simulink model "mac_simulink"  (R2025b)
settings: Solver=VariableStepAuto  StartTime=0.0  StopTime=39  RelTol=1e-3
libraries: hdlsllib x8
settings Model: Creator=aherrman  LastModifiedBy=aherrman

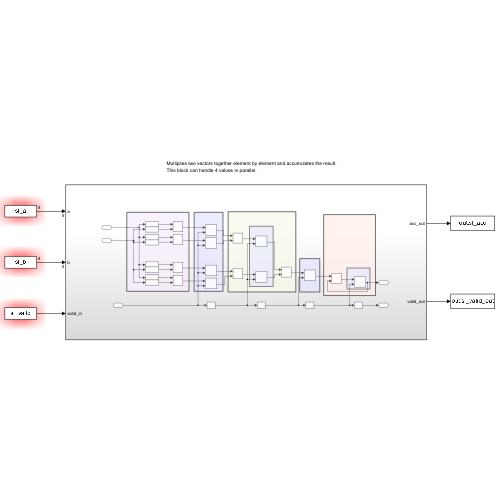
[thumbnail: Simulink's stored preview of the top-level diagram]
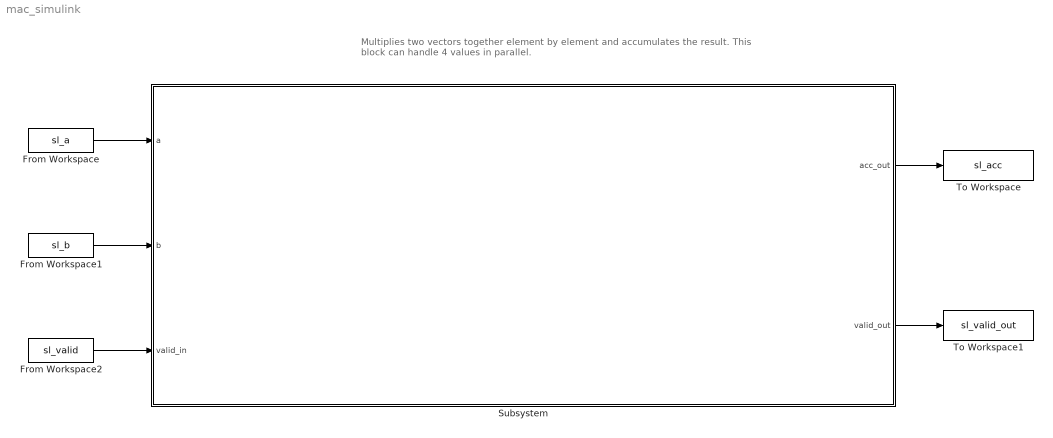
== system mac_simulink ==
  note: Multiplies two vectors together element by element and accumulates the result.
      | This block can handle 4 values in parallel.
  From Workspace : FromWorkspace  VariableName=sl_a  SampleTime=1  OutputAfterFinalValue=Setting to zero
  From Workspace1 : FromWorkspace  VariableName=sl_b  SampleTime=1  OutputAfterFinalValue=Setting to zero
  From Workspace2 : FromWorkspace  VariableName=sl_valid  SampleTime=1  OutputAfterFinalValue=Setting to zero
  Subsystem : Subsystem
  To Workspace : ToWorkspace  VariableName=sl_acc  SaveFormat=Timeseries  SampleTime=-1
  To Workspace1 : ToWorkspace  VariableName=sl_valid_out  SaveFormat=Timeseries  SampleTime=-1
  wires:
  From Workspace/1 -> Subsystem/1(a)
  From Workspace1/1 -> Subsystem/2(b)
  Subsystem/1(acc_out) -> To Workspace/1
  Subsystem/2(valid_out) -> To Workspace1/1
  From Workspace2/1 -> Subsystem/3(valid_in)

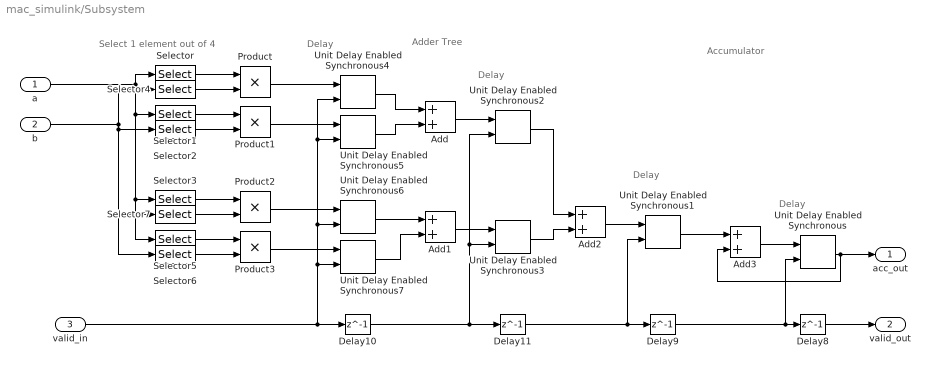
== system mac_simulink/Subsystem ==
  note: Accumulator
  note: Adder Tree
  note: Select 1 element
      | out of 4
  note: Delay
  note: Delay
  note: Delay
  note: Delay
  a : Inport
  b : Inport  Port=2
  valid_in : Inport  Port=3
  Add{,1..3} (4 alike) : Sum
  Delay{8..11} (4 alike) : Delay  DelayLength=1
  Product{,1..3} (4 alike) : Product
  Selector : Selector  IndexMode=Zero-based  InputPortWidth=4  IndexOptions=Index vector (dialog)  Indices=[0]  OutputSizes=1
  Selector1 : Selector  IndexMode=Zero-based  InputPortWidth=4  IndexOptions=Index vector (dialog)  Indices=[1]  OutputSizes=1
  Selector2 : Selector  IndexMode=Zero-based  InputPortWidth=4  IndexOptions=Index vector (dialog)  Indices=[1]  OutputSizes=1
  Selector3 : Selector  IndexMode=Zero-based  InputPortWidth=4  IndexOptions=Index vector (dialog)  Indices=[2]  OutputSizes=1
  Selector4 : Selector  IndexMode=Zero-based  InputPortWidth=4  IndexOptions=Index vector (dialog)  Indices=[0]  OutputSizes=1
  Selector5 : Selector  IndexMode=Zero-based  InputPortWidth=4  IndexOptions=Index vector (dialog)  Indices=[3]  OutputSizes=1
  Selector6 : Selector  IndexMode=Zero-based  InputPortWidth=4  IndexOptions=Index vector (dialog)  Indices=[3]  OutputSizes=1
  Selector7 : Selector  IndexMode=Zero-based  InputPortWidth=4  IndexOptions=Index vector (dialog)  Indices=[2]  OutputSizes=1
  Unit Delay Enabled Synchronous{,1..7} (8 alike) : hdlsllib/Discrete/Unit Delay Enabled Synchronous  InitialCondition=0.0  SampleTime=-1
  acc_out : Outport
  valid_out : Outport  Port=2
  wires:
  Selector5/1 -> Product3/1
  Unit Delay Enabled Synchronous1/1 -> Add3/1
  Unit Delay Enabled Synchronous6/1 -> Add1/1
  b/1 -> Selector6/1, Selector7/1, Selector2/1, Selector4/1
  Add/1 -> Unit Delay Enabled Synchronous2/1
  Unit Delay Enabled Synchronous/1 -> Add3/2, acc_out/1
  a/1 -> Selector5/1, Selector3/1, Selector1/1, Selector/1
  Selector/1 -> Product/1
  Selector2/1 -> Product1/2
  Add1/1 -> Unit Delay Enabled Synchronous3/1
  Unit Delay Enabled Synchronous7/1 -> Add1/2
  Add3/1 -> Unit Delay Enabled Synchronous/1
  Unit Delay Enabled Synchronous5/1 -> Add/2
  Selector1/1 -> Product1/1
  Add2/1 -> Unit Delay Enabled Synchronous1/1
  Selector7/1 -> Product2/2
  Selector6/1 -> Product3/2
  Unit Delay Enabled Synchronous4/1 -> Add/1
  Selector4/1 -> Product/2
  Selector3/1 -> Product2/1
  Delay8/1 -> valid_out/1
  Delay9/1 -> Unit Delay Enabled Synchronous/2, Delay8/1
  valid_in/1 -> Unit Delay Enabled Synchronous4/2, Unit Delay Enabled Synchronous5/2, Unit Delay Enabled Synchronous6/2, Unit Delay Enabled Synchronous7/2, Delay10/1
  Delay10/1 -> Unit Delay Enabled Synchronous2/2, Unit Delay Enabled Synchronous3/2, Delay11/1
  Delay11/1 -> Unit Delay Enabled Synchronous1/2, Delay9/1
  Unit Delay Enabled Synchronous3/1 -> Add2/2
  Unit Delay Enabled Synchronous2/1 -> Add2/1
  Product/1 -> Unit Delay Enabled Synchronous4/1
  Product1/1 -> Unit Delay Enabled Synchronous5/1
  Product2/1 -> Unit Delay Enabled Synchronous6/1
  Product3/1 -> Unit Delay Enabled Synchronous7/1
